simulink model "my_cart_pend"  (R2023b)
settings: Solver=ode4  StartTime=0.0  StopTime=20  FixedStep=0.001  RelTol=1e-3
values from neighbouring files (symbols this model uses):
  E_up = m*g*L*cos(0)    [init_HAC_simulation.m]    (also in init_model.m)
  eta = 1.3    [init_HAC_simulation.m]    (also in init_model.m)
  Fc = 0.00040    (= 0.0004)    [MPC_casadi_block.m]    (also in continuous_cartpend.m; init_HAC_simulation.m; init_MPC.m; init_NMPC.m)
  g = [g; st_next - st_next_RK4]    [MPC_cartPend_casadi.m]    (also in MPC_cartPend_casadi_scaled.m; MPC_casadi_block.m; continuous_cartpend.m = 9.80665; init_HAC_simulation.m = 9.80665)
  I = 8.7395e-04    (= 0.00087395)    [MPC_casadi_block.m]    (also in continuous_cartpend.m = 0.0008739525; init_HAC_simulation.m = 0.0008739525; init_MPC.m = 0.0008739525; init_NMPC.m = 0.0008739525)
  init_angle = 180    [MPC_cartPend_casadi.m]    (also in init_HAC_simulation.m = deg2rad(initial_angle); init_MPC.m = -0.349065850399; init_NMPC.m = 3.14159265359; init_PID_cartpole.m = 0)
  k_cw = 6    [init_HAC_simulation.m]    (also in init_model.m)
  k_em = 10    [init_HAC_simulation.m]    (also in init_model.m)
  k_lqr = discrete_lqr(m, M, L, I, g, kd, kt, Fc)    [init_HAC_simulation.m]    (also in init_model.m)
  k_su = 2    [init_HAC_simulation.m]    (also in init_model.m)
  k_vw = 2.5    [init_HAC_simulation.m]    (also in init_model.m)
  kd = 0.000161    [MPC_casadi_block.m]    (also in continuous_cartpend.m; init_HAC_simulation.m; init_MPC.m; init_NMPC.m)
  kdr = 0.000001    (= 1e-06)    [MPC_casadi_block.m]    (also in continuous_cartpend.m; init_HAC_simulation.m; init_MPC.m; init_NMPC.m)
  kt = 150    [MPC_casadi_block.m]    (also in continuous_cartpend.m; init_HAC_simulation.m; init_MPC.m; init_NMPC.m)
  L = 0.1500    (= 0.15)    [MPC_casadi_block.m]    (also in continuous_cartpend.m; init_HAC_simulation.m; init_MPC.m; init_NMPC.m)
  m = 0.116527    [MPC_casadi_block.m]    (also in continuous_cartpend.m; init_HAC_simulation.m; init_MPC.m; init_NMPC.m)
  uMax = 3*g    (= 29.41995)    [init_HAC_simulation.m]    (also in init_MPC.m; init_NMPC.m; init_model.m)
  x1_max = 0.43    [init_HAC_simulation.m]    (also in init_MPC.m; init_NMPC.m; init_model.m)
  x2_max = 2    [init_HAC_simulation.m]    (also in init_MPC.m; init_NMPC.m; init_model.m)
libraries: simulink_extras x2
settings Model: Creator=doann  LastModifiedBy=doann
settings OptimizationCC: ReuseModelBlockBuffer=off

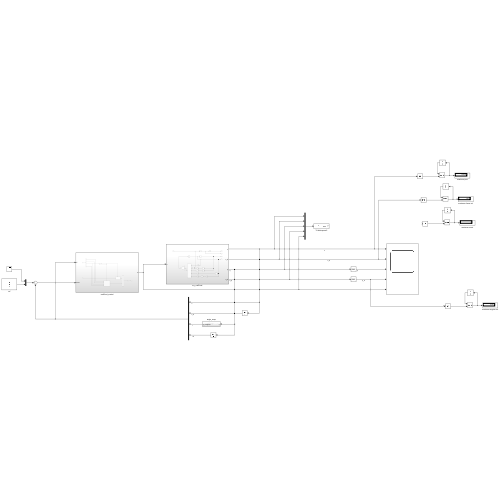
[thumbnail: Simulink's stored preview of the top-level diagram]
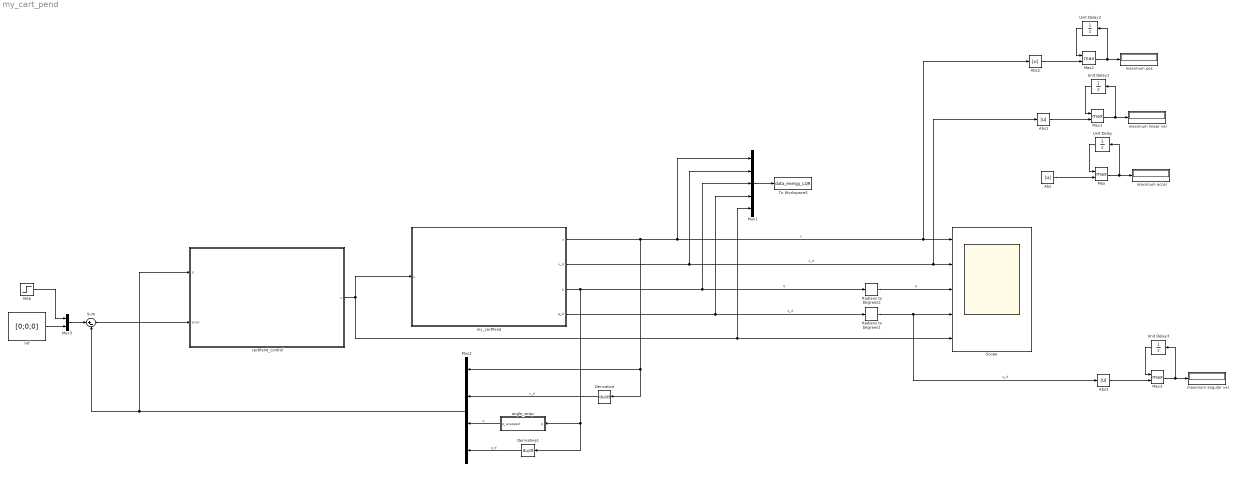
== system my_cart_pend ==
  Abs{,1..3} (4 alike) : Abs  SaturateOnIntegerOverflow=off
  Derivative : Derivative
  Derivative1 : Derivative
  Max{,1..3} (4 alike) : MinMax  Function=max  Inputs=2
  Mux1 : Mux  Inputs=5
  Mux2 : Mux
  Mux3 : Mux  Inputs=2
  Radians to Degrees1 : simulink_extras/Transformations/Radians to Degrees
  Radians to Degrees2 : simulink_extras/Transformations/Radians to Degrees
  Scope : Scope  NumInputPorts=5
  Step : Step  Time=10  After=0  SampleTime=0
  Sum : Sum  Inputs=|+-
  To Workspace5 : ToWorkspace  VariableName=data_energy_LQR  SaveFormat=Timeseries  SampleTime=-1
  Unit Delay{,1..3} (4 alike) : UnitDelay  SampleTime=-1  HasFrameUpgradeWarning=on
  angle_wrap : Subsystem
  cartPend_control : Subsystem  SystemSampleTime=0.001
  maximum accel : Display
  maximum angular vel : Display
  maximum linear vel : Display
  maximum pos : Display
  my_cartPend : Subsystem
  ref : Constant  Value=[0;0;0]  VectorParams1D=off
  wires:
  my_cartPend/4(q_d) -> Radians to Degrees1/1, Mux1/4  "q_d"
  my_cartPend/3(q) -> Derivative1/1, angle_wrap/1(q), Radians to Degrees2/1, Mux1/3  "q"
  angle_wrap/1(q_wrapped) -> Mux2/3  "q"
  Mux3/1 -> Sum/1
  Radians to Degrees2/1 -> Scope/3  "q"
  Abs/1 -> Max/2
  Max/1 -> Unit Delay/1, maximum accel/1
  Unit Delay/1 -> Max/1
  Unit Delay1/1 -> Max1/1
  Max1/1 -> maximum linear vel/1, Unit Delay1/1
  Abs1/1 -> Max1/2
  my_cartPend/2(x_d) -> Abs1/1, Scope/2, Mux1/2  "x_d"
  my_cartPend/1(x) -> Derivative/1, Mux2/1, Mux1/1, Abs2/1, Scope/1  "x"
  Abs2/1 -> Max2/2
  Max2/1 -> Unit Delay2/1, maximum pos/1
  Unit Delay2/1 -> Max2/1
  Mux2/1 -> cartPend_control/1(X), Sum/2
  Derivative/1 -> Mux2/2  "x_d"
  Derivative1/1 -> Mux2/4  "q_d"
  Unit Delay3/1 -> Max3/1
  Max3/1 -> maximum angular vel/1, Unit Delay3/1
  Abs3/1 -> Max3/2
  Radians to Degrees1/1 -> Abs3/1, Scope/4  "q_d"
  Mux1/1 -> To Workspace5/1
  Step/1 -> Mux3/1
  ref/1 -> Mux3/2
  Sum/1 -> cartPend_control/2(error)
  cartPend_control/1(u) -> Mux1/5, Scope/5, my_cartPend/1(u)

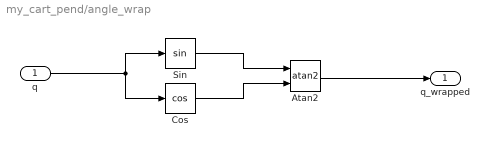
== system my_cart_pend/angle_wrap ==
  q : Inport
  Atan2 : Trigonometry  Operator=atan2
  Cos : Trigonometry  Operator=cos
  Sin : Trigonometry
  q_wrapped : Outport
  wires:
  Cos/1 -> Atan2/2
  q/1 -> Sin/1, Cos/1
  Sin/1 -> Atan2/1
  Atan2/1 -> q_wrapped/1

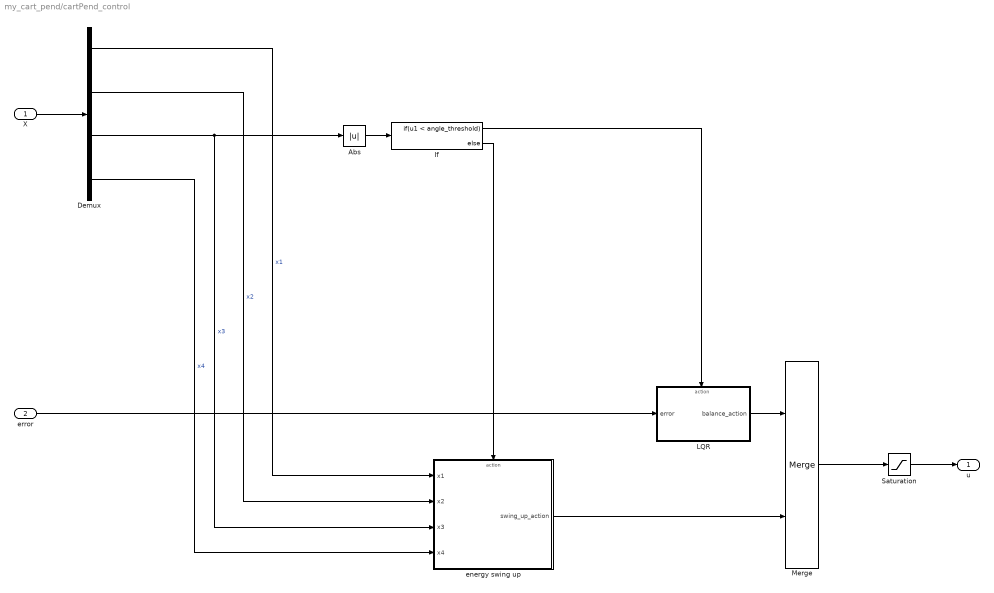
== system my_cart_pend/cartPend_control ==
  X : Inport
  error : Inport  Port=2
  Abs : Abs  SaturateOnIntegerOverflow=off
  Demux : Demux
  If : If  IfExpression=u1 < angle_threshold
  LQR : Subsystem  TreatAsAtomicUnit=on
  Merge : Merge
  Saturation : Saturate  UpperLimit=uMax  LowerLimit=-uMax
  energy swing up : Subsystem  TreatAsAtomicUnit=on
  u : Outport
  wires:
  X/1 -> Demux/1
  Demux/3 -> Abs/1, energy swing up/3(x3)  "x3"
  Demux/4 -> energy swing up/4(x4)  "x4"
  Abs/1 -> If/1
  If/1 -> LQR/Action
  If/2 -> energy swing up/Action
  LQR/1(balance_action) -> Merge/1
  energy swing up/1(swing_up_action) -> Merge/2
  error/1 -> LQR/1(error)
  Demux/2 -> energy swing up/2(x2)  "x2"
  Demux/1 -> energy swing up/1(x1)  "x1"
  Merge/1 -> Saturation/1
  Saturation/1 -> u/1

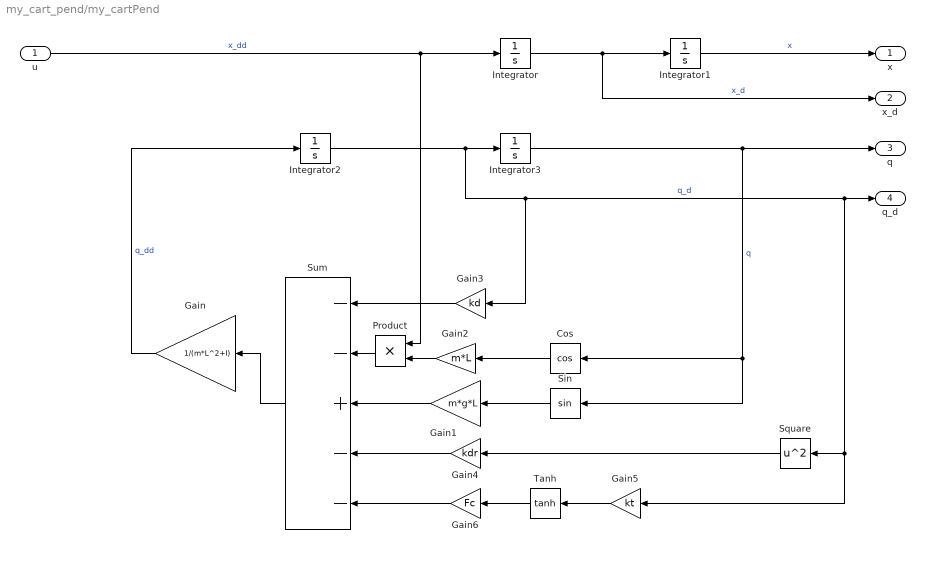
== system my_cart_pend/my_cartPend ==
  u : Inport
  Cos : Trigonometry  Operator=cos
  Gain : Gain  Gain=1/(m*L^2+I)
  Gain1 : Gain  Gain=m*g*L
  Gain2 : Gain  Gain=m*L
  Gain3 : Gain  Gain=kd
  Gain4 : Gain  Gain=kdr
  Gain5 : Gain  Gain=kt
  Gain6 : Gain  Gain=Fc
  Integrator : Integrator
  Integrator1 : Integrator
  Integrator2 : Integrator
  Integrator3 : Integrator  InitialCondition=init_angle
  Product : Product
  Sin : Trigonometry
  Square : Math  Operator=square
  Sum : Sum  Inputs=--+--
  Tanh : Trigonometry  Operator=tanh
  x : Outport
  x_d : Outport  Port=2
  q : Outport  Port=3
  q_d : Outport  Port=4
  wires:
  u/1 -> Product/1, Integrator/1  "x_dd"
  Integrator/1 -> x_d/1, Integrator1/1  "x_d"
  Integrator1/1 -> x/1  "x"
  Integrator3/1 -> Sin/1, Cos/1, q/1  "q"
  Integrator2/1 -> Gain3/1, Gain5/1, Square/1, q_d/1, Integrator3/1  "q_d"
  Sin/1 -> Gain1/1
  Cos/1 -> Gain2/1
  Sum/1 -> Gain/1
  Gain/1 -> Integrator2/1  "q_dd"
  Gain1/1 -> Sum/3
  Gain3/1 -> Sum/1
  Gain2/1 -> Product/2
  Product/1 -> Sum/2
  Square/1 -> Gain4/1
  Tanh/1 -> Gain6/1
  Gain5/1 -> Tanh/1
  Gain4/1 -> Sum/4
  Gain6/1 -> Sum/5

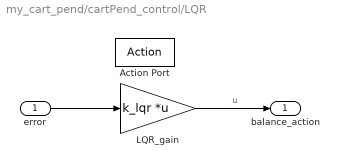
== system my_cart_pend/cartPend_control/LQR ==
  error : Inport
  Action Port : ActionPort  ActionPortLabel=if(u1 < angle_threshold)
  LQR_gain : Gain  Gain=k_lqr  Multiplication=Matrix(K*u)
  balance_action : Outport
  wires:
  error/1 -> LQR_gain/1
  LQR_gain/1 -> balance_action/1  "u"

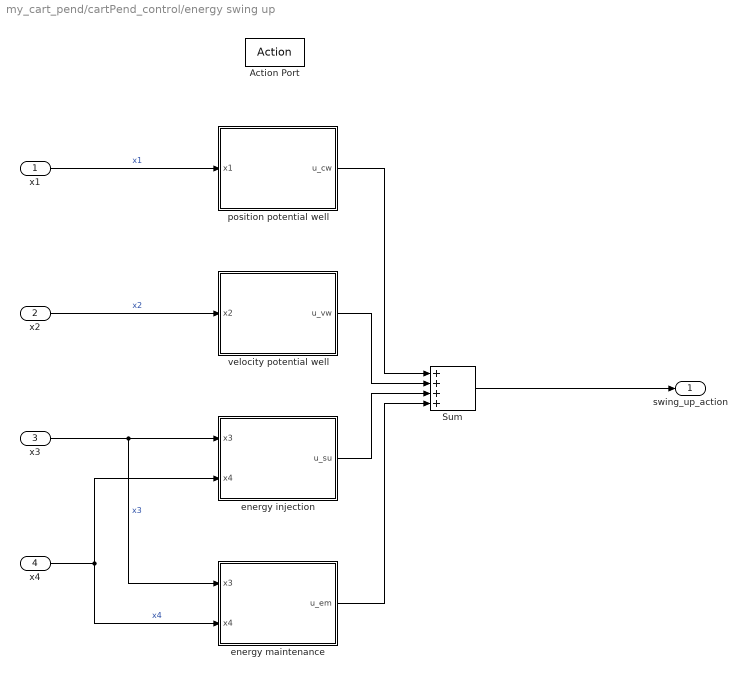
== system my_cart_pend/cartPend_control/energy swing up ==
  x1 : Inport
  x2 : Inport  Port=2
  x3 : Inport  Port=3
  x4 : Inport  Port=4
  Action Port : ActionPort  ActionPortLabel=else
  Sum : Sum  Inputs=++++
  energy injection : Subsystem
  energy maintenance : Subsystem
  position potential well : Subsystem
  velocity potential well : Subsystem
  swing_up_action : Outport
  wires:
  energy injection/1(u_su) -> Sum/3
  x2/1 -> velocity potential well/1(x2)  "x2"
  velocity potential well/1(u_vw) -> Sum/2
  Sum/1 -> swing_up_action/1
  energy maintenance/1(u_em) -> Sum/4
  x3/1 -> energy maintenance/1(x3), energy injection/1(x3)  "x3"
  x1/1 -> position potential well/1(x1)  "x1"
  x4/1 -> energy injection/2(x4), energy maintenance/2(x4)  "x4"
  position potential well/1(u_cw) -> Sum/1

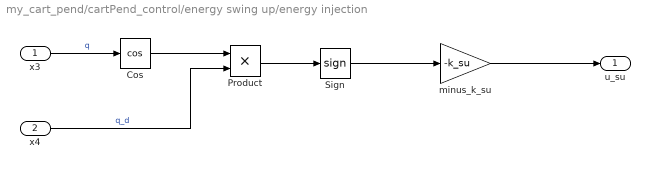
== system my_cart_pend/cartPend_control/energy swing up/energy injection ==
  x3 : Inport
  x4 : Inport  Port=2
  Cos : Trigonometry  Operator=cos
  Product : Product
  Sign : Signum
  minus_k_su : Gain  Gain=-k_su
  u_su : Outport
  wires:
  x3/1 -> Cos/1  "q"
  x4/1 -> Product/2  "q_d"
  Sign/1 -> minus_k_su/1
  minus_k_su/1 -> u_su/1
  Cos/1 -> Product/1
  Product/1 -> Sign/1

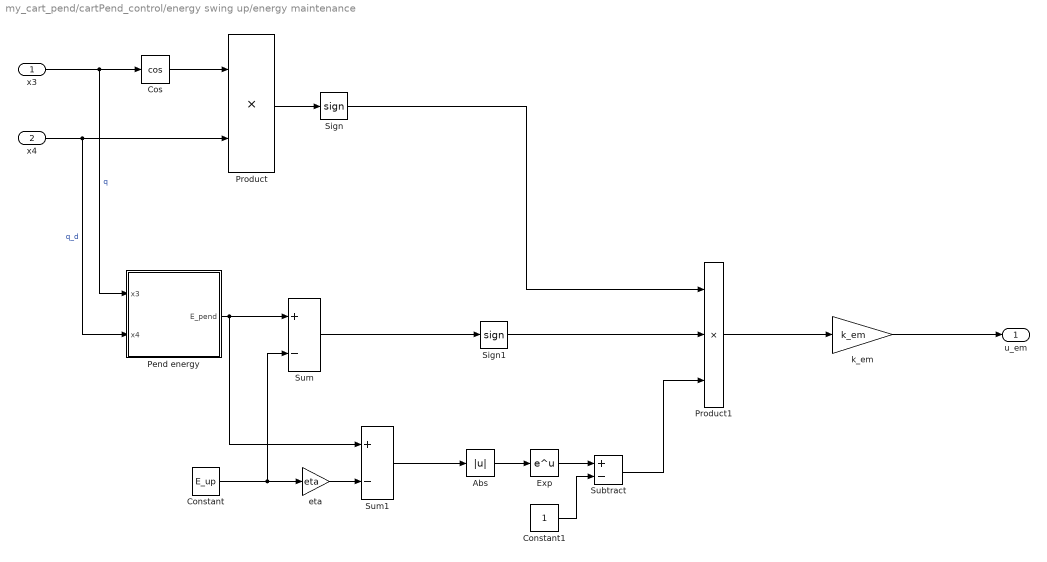
== system my_cart_pend/cartPend_control/energy swing up/energy maintenance ==
  x3 : Inport
  x4 : Inport  Port=2
  Abs : Abs  SaturateOnIntegerOverflow=off
  Constant : Constant  Value=E_up
  Constant1 : Constant
  Cos : Trigonometry  Operator=cos
  Exp : Math
  Pend energy : Subsystem
  Product : Product
  Product1 : Product  Inputs=3
  Sign : Signum
  Sign1 : Signum
  Subtract : Sum  Inputs=+-
  Sum : Sum  Inputs=+-
  Sum1 : Sum  Inputs=+-
  eta : Gain  Gain=eta
  k_em : Gain  Gain=k_em
  u_em : Outport
  wires:
  x3/1 -> Pend energy/1(x3), Cos/1  "q"
  Cos/1 -> Product/1
  x4/1 -> Pend energy/2(x4), Product/2  "q_d"
  Product/1 -> Sign/1
  Pend energy/1(E_pend) -> Sum/1, Sum1/1
  Constant/1 -> Sum/2, eta/1
  Sum/1 -> Sign1/1
  eta/1 -> Sum1/2
  Sum1/1 -> Abs/1
  Abs/1 -> Exp/1
  Exp/1 -> Subtract/1
  Constant1/1 -> Subtract/2
  Sign1/1 -> Product1/2
  Sign/1 -> Product1/1
  Subtract/1 -> Product1/3
  Product1/1 -> k_em/1
  k_em/1 -> u_em/1

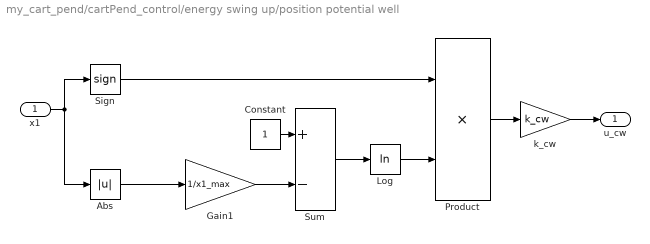
== system my_cart_pend/cartPend_control/energy swing up/position potential well ==
  x1 : Inport
  Abs : Abs  SaturateOnIntegerOverflow=off
  Constant : Constant
  Gain1 : Gain  Gain=1/x1_max
  Log : Math  Operator=log
  Product : Product
  Sign : Signum
  Sum : Sum  Inputs=+-
  k_cw : Gain  Gain=k_cw
  u_cw : Outport
  wires:
  x1/1 -> Abs/1, Sign/1
  Abs/1 -> Gain1/1
  Gain1/1 -> Sum/2
  Constant/1 -> Sum/1
  Sum/1 -> Log/1
  k_cw/1 -> u_cw/1
  Product/1 -> k_cw/1
  Log/1 -> Product/2
  Sign/1 -> Product/1

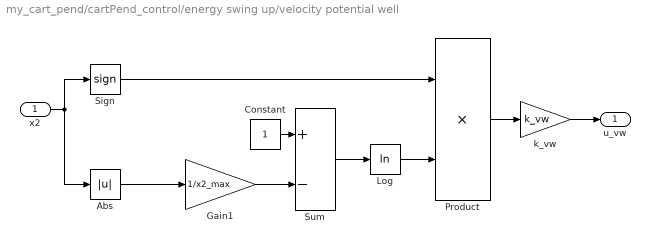
== system my_cart_pend/cartPend_control/energy swing up/velocity potential well ==
  x2 : Inport
  Abs : Abs  SaturateOnIntegerOverflow=off
  Constant : Constant
  Gain1 : Gain  Gain=1/x2_max
  Log : Math  Operator=log
  Product : Product
  Sign : Signum
  Sum : Sum  Inputs=+-
  k_vw : Gain  Gain=k_vw
  u_vw : Outport
  wires:
  Sign/1 -> Product/1
  Log/1 -> Product/2
  Product/1 -> k_vw/1
  k_vw/1 -> u_vw/1
  Sum/1 -> Log/1
  Constant/1 -> Sum/1
  Gain1/1 -> Sum/2
  Abs/1 -> Gain1/1
  x2/1 -> Sign/1, Abs/1

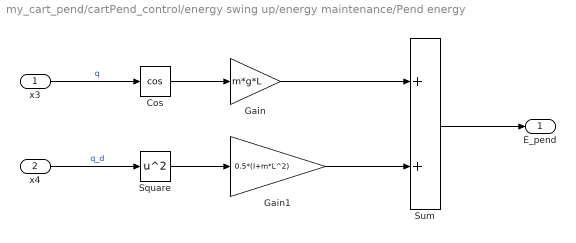
== system my_cart_pend/cartPend_control/energy swing up/energy maintenance/Pend energy ==
  x3 : Inport
  x4 : Inport  Port=2
  Cos : Trigonometry  Operator=cos
  Gain : Gain  Gain=m*g*L
  Gain1 : Gain  Gain=0.5*(I+m*L^2)
  Square : Math  Operator=square
  Sum : Sum
  E_pend : Outport
  wires:
  x3/1 -> Cos/1  "q"
  x4/1 -> Square/1  "q_d"
  Cos/1 -> Gain/1
  Square/1 -> Gain1/1
  Gain/1 -> Sum/1
  Gain1/1 -> Sum/2
  Sum/1 -> E_pend/1
